simulink model "controladaptable"  (R2023b)
settings: Solver=ode23t  StartTime=0.0  StopTime=25  RelTol=1e-3
values from neighbouring files (symbols this model uses):
  BL = 0.00223579    [ILCadaptable.m]    (also in parametros3.m)
  C1 = [1 0 0 0]    [ILCadaptable.m]    (also in parametros3.m = [1 0 0 0 0 0])
  C2 = [0 1 0 0]    [ILCadaptable.m]    (also in parametros3.m = [0 0 1 0 0 0])
  C3 = [0 0 1 0]    [ILCadaptable.m]    (also in parametros3.m = [0 0 0 0 1 0])
  C4 = [0 0 0 1]    [ILCadaptable.m]
  JL = 0.00040095    [ILCadaptable.m]    (also in parametros3.m)
  KB = 0.23351629    [ILCadaptable.m]    (also in parametros3.m)
  KD = 5    [ILCadaptable.m]
  KM = 0.23351629    [ILCadaptable.m]    (also in parametros3.m)
  LC = 0.0015    [ILCadaptable.m]    (also in parametros3.m)
  RC = 3.4    [ILCadaptable.m]    (also in parametros3.m)
  rt = 10    [ILCadaptable.m]    (also in parametros3.m)
libraries: simulink x2, slpidlib x2
settings Model: Creator=soria  LastModifiedBy=LENOVO
settings SolverCC: AlgebraicLoopSolver=TrustRegion
settings DebuggingCC: UnconnectedInputMsg=warning  UnconnectedOutputMsg=warning  UnconnectedLineMsg=warning
settings ModelReferenceCC: EnableRefExpFcnMdlSchedulingChecks=on

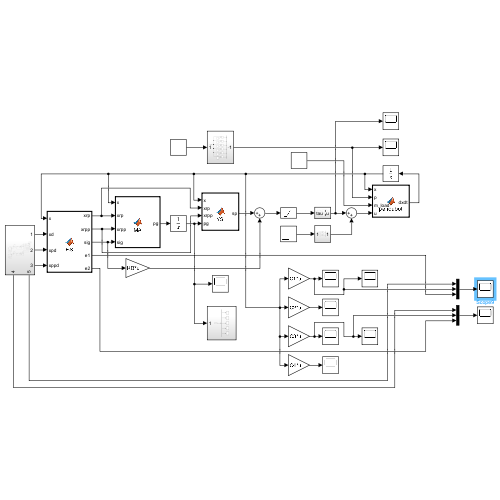
[thumbnail: Simulink's stored preview of the top-level diagram]
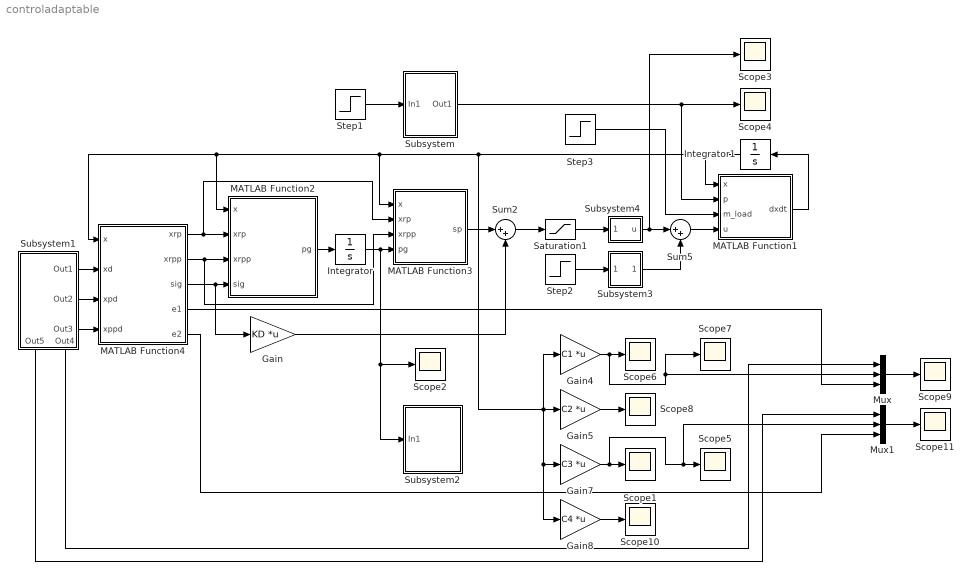
== system controladaptable ==
  Gain : Gain  Gain=KD  Multiplication=Matrix(K*u)
  Gain4 : Gain  Gain=C1  Multiplication=Matrix(K*u)
  Gain5 : Gain  Gain=C2  Multiplication=Matrix(K*u)
  Gain7 : Gain  Gain=C3  Multiplication=Matrix(K*u)
  Gain8 : Gain  Gain=C4  Multiplication=Matrix(K*u)
  Integrator : Integrator  InitialCondition=[0 0 0 0 0]
  Integrator1 : Integrator  InitialCondition=[-pi/2;0;0;0]
  MATLAB Function1 : MATLAB Function  TreatAsAtomicUnit=on
  MATLAB Function2 : MATLAB Function  TreatAsAtomicUnit=on
  MATLAB Function3 : MATLAB Function  TreatAsAtomicUnit=on
  MATLAB Function4 : MATLAB Function  TreatAsAtomicUnit=on
  Mux : Mux  Inputs=3
  Mux1 : Mux  Inputs=3
  Saturation1 : Saturate  UpperLimit=10  LowerLimit=-10
  Scope{1..11} (11 alike) : Scope
  Step1 : Step  Time=0  SampleTime=0
  Step2 : Step  Time=0  After=2  SampleTime=0
  Step3 : Step  Time=10  SampleTime=0
  Subsystem : Subsystem
  Subsystem1 : Subsystem
      settings: PortSchema="{\"entries\":[{\"content\":{\"sides\":[{\"content\":{},\"type\":\"ConnectorPlacement.EquallySpacedRectSide\",\"uuid\":\"9b7d0a68-027c-45ca-820c-f278bc6f32a7\"},{\"content\":{\"connectorIds\":[\"Out1\",\"Out2\",\"Out3\"],\"side\":\"RIGHT\"},\"type\":\"ConnectorPlacement.EquallySpacedRectSide\",\"uuid\":\"fa53ec67-4df6-4868-87ee-3d32a2fc1068\"},{\"content\":{\"side\":\"TOP\"},\"type\":\"ConnectorPlacement.EquallySpacedRectSide\",\"uuid\":\"8fcd41cb-9cc9-4cf7-b08f-50ea27c8effa\"},{\"content\":{\"connectorIds\":[\"Out4\",\"Out5\"],\"side\":\"BOTTOM\"},\"type\":\"ConnectorPlacement.EquallySpacedRectSide\",\"uuid\":\"53ef6b28-bc02-4c26-b41f-4cbf5a6224bd\"}]},\"type\":\"ConnectorPlacement.EquallySpacedConnector\",\"uuid\":\"01489902-74b8-4eba-a27b-b5ca226e6d88\"}],\"packageUris\":[\"http://schema.mathworks.com/mf0/Connector/R2020b\"],\"version\":\"1.0\"}"
  Subsystem2 : Subsystem
  Subsystem3 : Subsystem
  Subsystem4 : Subsystem
  Sum2 : Sum  Inputs=|++
  Sum5 : Sum  Inputs=|++
  wires:
  MATLAB Function2/1(pg) -> Integrator/1
  MATLAB Function4/3(sig) -> Gain/1, MATLAB Function2/4(sig)
  Gain4/1 -> Scope7/1, Mux/2, Scope6/1
  Gain7/1 -> Scope5/1, Mux1/2, Scope1/1
  Gain5/1 -> Scope8/1
  Gain8/1 -> Scope10/1
  MATLAB Function4/2(xrpp) -> MATLAB Function2/3(xrpp), MATLAB Function3/3(xrpp)
  Subsystem1/3(Out3) -> MATLAB Function4/4(xppd)
  Subsystem1/1(Out1) -> MATLAB Function4/2(xd)
  Subsystem1/2(Out2) -> MATLAB Function4/3(xpd)
  Step1/1 -> Subsystem/1(In1)
  Integrator/1 -> Subsystem2/1(In1), Scope2/1, MATLAB Function3/4(pg)
  Integrator1/1 -> MATLAB Function1/1(x), Gain4/1, Gain8/1, Gain7/1, Gain5/1, MATLAB Function2/1(x), MATLAB Function4/1(x), MATLAB Function3/1(x)
  Subsystem/1(Out1) -> Scope4/1, MATLAB Function1/2(p)
  MATLAB Function3/1(sp) -> Sum2/1
  MATLAB Function4/1(xrp) -> MATLAB Function3/2(xrp), MATLAB Function2/2(xrp)
  MATLAB Function1/1(dxdt) -> Integrator1/1
  Mux/1 -> Scope9/1
  Mux1/1 -> Scope11/1
  Subsystem1/5(Out4) -> Mux/1
  Subsystem1/4(Out5) -> Mux1/1
  Subsystem3/1(Out1) -> Sum5/2
  Step2/1 -> Subsystem3/1(In1)
  Gain/1 -> Sum2/2
  Sum5/1 -> MATLAB Function1/4(u)
  Subsystem4/1(u) -> Scope3/1, Sum5/1
  MATLAB Function4/4(e1) -> Mux/3
  MATLAB Function4/5(e2) -> Mux1/3
  Sum2/1 -> Saturation1/1
  Saturation1/1 -> Subsystem4/1(tau)
  Step3/1 -> MATLAB Function1/3(m_load)

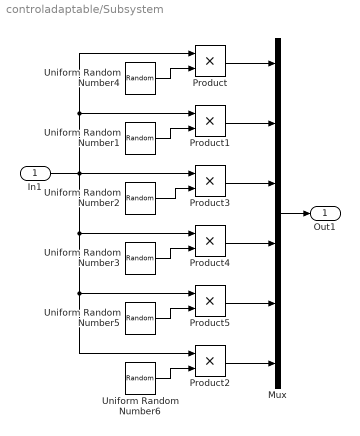
== system controladaptable/Subsystem ==
  In1 : Inport
  Mux : Mux  Inputs=6
  Product{,1..5} (6 alike) : Product
  Uniform Random Number1 : UniformRandomNumber  Minimum=-0.0792  Maximum=0.0792  Seed=2  SampleTime=0.1
  Uniform Random Number2 : UniformRandomNumber  Minimum=-0.025  Maximum=0.025  Seed=1  SampleTime=0.1
  Uniform Random Number3 : UniformRandomNumber  Minimum=-0.03  Maximum=0.03  Seed=3  SampleTime=0.1
  Uniform Random Number4 : UniformRandomNumber  Minimum=-0.066  Maximum=0.066  SampleTime=0.1
  Uniform Random Number5 : UniformRandomNumber  Minimum=-0.00138  Maximum=0.00138  Seed=1.5  SampleTime=0.1
  Uniform Random Number6 : UniformRandomNumber  Minimum=-0.00238  Maximum=0.00238  Seed=1.5  SampleTime=0.1
  Out1 : Outport
  wires:
  Product/1 -> Mux/1
  Uniform Random Number5/1 -> Product5/2
  Uniform Random Number1/1 -> Product1/2
  In1/1 -> Product2/1, Product5/1, Product4/1, Product3/1, Product/1, Product1/1
  Uniform Random Number2/1 -> Product3/2
  Product4/1 -> Mux/4
  Product1/1 -> Mux/2
  Uniform Random Number3/1 -> Product4/2
  Uniform Random Number4/1 -> Product/2
  Product3/1 -> Mux/3
  Product5/1 -> Mux/5
  Mux/1 -> Out1/1
  Product2/1 -> Mux/6
  Uniform Random Number6/1 -> Product2/2

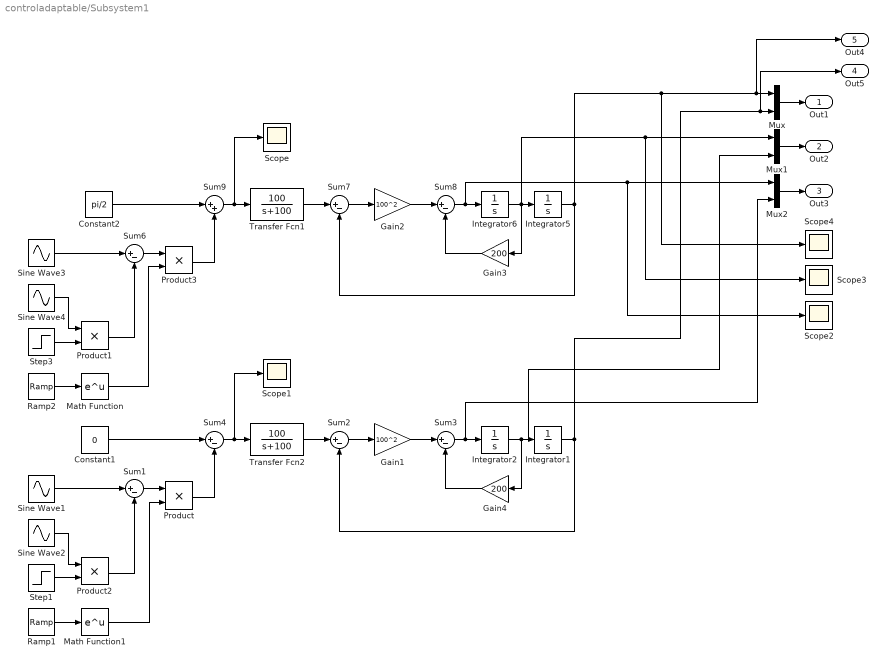
== system controladaptable/Subsystem1 ==
  Constant1 : Constant  Value=0
  Constant2 : Constant  Value=pi/2
  Gain1 : Gain  Gain=100^2
  Gain2 : Gain  Gain=100^2
  Gain3 : Gain  Gain=200
  Gain4 : Gain  Gain=200
  Integrator{1..2,5..6} (4 alike) : Integrator
  Math Function : Math
  Math Function1 : Math
  Mux : Mux  Inputs=2
  Mux1 : Mux  Inputs=2
  Mux2 : Mux  Inputs=2
  Product{,1..3} (4 alike) : Product
  Ramp1 : simulink/Sources/Ramp  slope=0  start=10  InitialOutput=0
  Ramp2 : simulink/Sources/Ramp  slope=0  start=10  InitialOutput=0
  Scope{,1..4} (5 alike) : Scope
  Sine Wave1 : Sin  Amplitude=1.4  Frequency=2  SampleTime=0
  Sine Wave2 : Sin  Amplitude=1.4  Frequency=5  SampleTime=0
  Sine Wave3 : Sin  Amplitude=1.4  Frequency=2  SampleTime=0
  Sine Wave4 : Sin  Amplitude=1.4  Frequency=5  SampleTime=0
  Step1 : Step  Time=0  After=0  SampleTime=0
  Step3 : Step  Time=0  After=0  SampleTime=0
  Sum{1..4,6..8} (7 alike) : Sum  Inputs=|+-
  Sum9 : Sum  Inputs=|++
  Transfer Fcn1 : TransferFcn  Numerator=[100]  Denominator=[1 100]
  Transfer Fcn2 : TransferFcn  Numerator=[100]  Denominator=[1 100]
  Out1 : Outport
  Out2 : Outport  Port=2
  Out3 : Outport  Port=3
  Out5 : Outport  Port=4
  Out4 : Outport  Port=5
  wires:
  Mux/1 -> Out1/1
  Mux1/1 -> Out2/1
  Mux2/1 -> Out3/1
  Integrator5/1 -> Scope4/1, Out4/1, Mux/1, Sum7/2
  Sine Wave3/1 -> Sum6/1
  Sum7/1 -> Gain2/1
  Sum8/1 -> Scope2/1, Mux2/1, Integrator6/1
  Sine Wave4/1 -> Product1/1
  Gain2/1 -> Sum8/1
  Transfer Fcn1/1 -> Sum7/1
  Gain3/1 -> Sum8/2
  Product1/1 -> Sum6/2
  Step3/1 -> Product1/2
  Constant2/1 -> Sum9/1
  Integrator6/1 -> Scope3/1, Mux1/1, Gain3/1, Integrator5/1
  Sum9/1 -> Scope/1, Transfer Fcn1/1
  Sum4/1 -> Scope1/1, Transfer Fcn2/1
  Sum3/1 -> Mux2/2, Integrator2/1
  Gain1/1 -> Sum3/1
  Transfer Fcn2/1 -> Sum2/1
  Sum2/1 -> Gain1/1
  Step1/1 -> Product2/2
  Constant1/1 -> Sum4/1
  Integrator1/1 -> Out5/1, Mux/2, Sum2/2
  Sine Wave1/1 -> Sum1/1
  Gain4/1 -> Sum3/2
  Integrator2/1 -> Mux1/2, Gain4/1, Integrator1/1
  Product2/1 -> Sum1/2
  Sine Wave2/1 -> Product2/1
  Math Function/1 -> Product3/2
  Math Function1/1 -> Product/2
  Ramp2/1 -> Math Function/1
  Ramp1/1 -> Math Function1/1
  Sum6/1 -> Product3/1
  Product3/1 -> Sum9/2
  Sum1/1 -> Product/1
  Product/1 -> Sum4/2

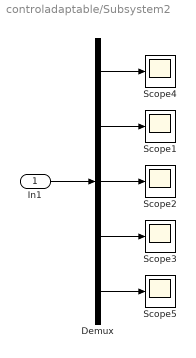
== system controladaptable/Subsystem2 ==
  In1 : Inport
  Demux : Demux  Outputs=5
  Scope{1..5} (5 alike) : Scope
  wires:
  In1/1 -> Demux/1
  Demux/3 -> Scope2/1
  Demux/2 -> Scope1/1
  Demux/1 -> Scope4/1
  Demux/4 -> Scope3/1
  Demux/5 -> Scope5/1

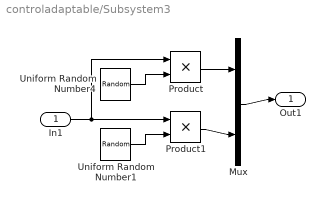
== system controladaptable/Subsystem3 ==
  In1 : Inport
  Mux : Mux  Inputs=2
  Product : Product
  Product1 : Product
  Uniform Random Number1 : UniformRandomNumber  Seed=2  SampleTime=0.1
  Uniform Random Number4 : UniformRandomNumber  SampleTime=0.1
  Out1 : Outport
  wires:
  Product/1 -> Mux/1
  Uniform Random Number1/1 -> Product1/2
  In1/1 -> Product/1, Product1/1
  Product1/1 -> Mux/2
  Uniform Random Number4/1 -> Product/2
  Mux/1 -> Out1/1

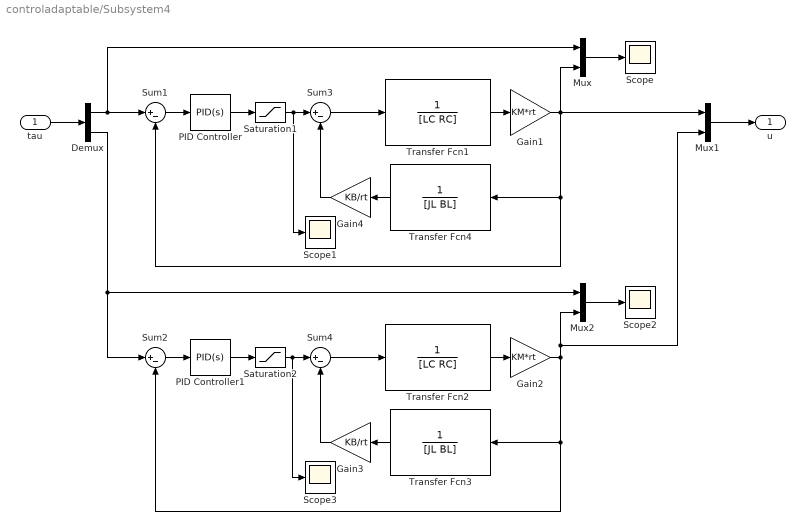
== system controladaptable/Subsystem4 ==
  tau : Inport
  Demux : Demux  Outputs=2
  Gain1 : Gain  Gain=KM*rt
  Gain2 : Gain  Gain=KM*rt
  Gain3 : Gain  Gain=KB/rt
  Gain4 : Gain  Gain=KB/rt
  Mux : Mux  Inputs=2
  Mux1 : Mux  Inputs=2
  Mux2 : Mux  Inputs=2
  PID Controller : slpidlib/PID Controller  Controller=PID  Form=Parallel  TimeDomain=Continuous-time  UseExternalTs=off  SampleTime=-1  IntegratorMethod=Forward Euler  FilterMethod=Forward Euler  ControllerParametersSource=internal  P=100  I=50  UseKiTs=off  D=20  N=100  UseFilter=on  TunerSelectOption=Transfer Function Based (PID Tuner App)  InitialConditionSource=internal  InitialConditionForIntegrator=0  InitialConditionForFilter=0  DifferentiatorICPrevScaledInput=0  ExternalReset=none  TrackingMode=off  Kt=1  LimitOutput=off  SatLimitsSource=internal  UpperSaturationLimit=inf  LowerSaturationLimit=-inf  LinearizeAsGain=on  AntiWindupMode=none  Kb=1  LimitIntegrator=off  UpperIntegratorSaturationLimit=inf  LowerIntegratorSaturationLimit=-inf  POutMin=[]  POutMax=[]  IOutMin=[]  IOutMax=[]  DOutMin=[]  DOutMax=[]  NOutMin=[]  NOutMax=[]  SumOutMin=[]  SumOutMax=[]  SaturationOutMin=[]  SaturationOutMax=[]  PParamMin=[]  PParamMax=[]  IParamMin=[]  IParamMax=[]  DParamMin=[]  DParamMax=[]  NParamMin=[]  NParamMax=[]  KbParamMin=[]  KbParamMax=[]  KtParamMin=[]  KtParamMax=[]  KbOutMin=[]  KbOutMax=[]  KtOutMin=[]  KtOutMax=[]  IntegratorOutMin=[]  IntegratorOutMax=[]  FilterOutMin=[]  FilterOutMax=[]  SumI1OutMin=[]  SumI1OutMax=[]  SumI2OutMin=[]  SumI2OutMax=[]  SumI3OutMin=[]  SumI3OutMax=[]  SumI4OutMin=[]  SumI4OutMax=[]  SumDOutMin=[]  SumDOutMax=[]  DifferentiatorOutMin=[]  DifferentiatorOutMax=[]  FilterDiffOutCoefMin=[]  FilterDiffOutCoefMax=[]  ReciprocalOutMin=[]  ReciprocalOutMax=[]  SumDenOutMin=[]  SumDenOutMax=[]  SumNumOutMin=[]  SumNumOutMax=[]  DivideOutMin=[]  DivideOutMax=[]  UdiffTsProdOutMin=[]  UdiffTsProdOutMax=[]  NTsProdOutMin=[]  NTsProdOutMax=[]  UintegralTsProdOutMin=[]  UintegralTsProdOutMax=[]  UngainTsProdOutMin=[]  UngainTsProdOutMax=[]  ClampingZeroOutDataTypeStr=Inherit: Inherit via back propagation  ClampingZeroOutMin=[]  ClampingZeroOutMax=[]  FilterDenConstantOutDataTypeStr=Inherit: Inherit via back propagation  FilterDenConstantOutMin=[]  FilterDenConstantOutMax=[]  PCopyOutDataTypeStr=Inherit: Inherit via back propagation  PCopyOutMin=[]  PCopyOutMax=[]  NCopyOutDataTypeStr=Inherit: Inherit via back propagation  NCopyOutMin=[]  NCopyOutMax=[]  IntegratorContinuousStateAttributes=''  IntegratorStateMustResolveToSignalObject=off  IntegratorRTWStateStorageClass=Auto  FilterContinuousStateAttributes=''  FilterStateMustResolveToSignalObject=off  FilterRTWStateStorageClass=Auto  ParallelPVariant=InternalParameters  IdealPVariant=Disabled  IVariant=InternalParameters  DVariant=InternalParameters  IntegratorVariant=Continuous  SatVariant=Disabled  AWVariant=Passthrough  PCopyVariant=Disabled  TRVariant=Disabled  FdbkBlocksVariant=Forward  IdealPFdbkVariant=Disabled  SatFdbkVariant=Disabled  DerivativeFilterVariant=ContFilter  NVariant=InternalParameters  NCopyVariant=Disabled  FilterICVariant=InternalICsFilter  IntegratorICVariant=InternalICs  ExternalResetVariant=Disabled  TRSumVariant=Passthrough  SumFdbkVariant=Disabled  SumVariant=Sum_PID  TsampFilterVariant=InternalTs  TsampNgainVariant=Passthrough  TsampIntegralVariant=Disabled_SignalSpec  ExternalSaturationOutDataTypeStr=Inherit: Same as second input
  PID Controller1 : slpidlib/PID Controller  Controller=PID  Form=Parallel  TimeDomain=Continuous-time  UseExternalTs=off  SampleTime=-1  IntegratorMethod=Forward Euler  FilterMethod=Forward Euler  ControllerParametersSource=internal  P=100  I=50  UseKiTs=off  D=20  N=100  UseFilter=on  TunerSelectOption=Transfer Function Based (PID Tuner App)  InitialConditionSource=internal  InitialConditionForIntegrator=0  InitialConditionForFilter=0  DifferentiatorICPrevScaledInput=0  ExternalReset=none  TrackingMode=off  Kt=1  LimitOutput=off  SatLimitsSource=internal  UpperSaturationLimit=inf  LowerSaturationLimit=-inf  LinearizeAsGain=on  AntiWindupMode=none  Kb=1  LimitIntegrator=off  UpperIntegratorSaturationLimit=inf  LowerIntegratorSaturationLimit=-inf  POutMin=[]  POutMax=[]  IOutMin=[]  IOutMax=[]  DOutMin=[]  DOutMax=[]  NOutMin=[]  NOutMax=[]  SumOutMin=[]  SumOutMax=[]  SaturationOutMin=[]  SaturationOutMax=[]  PParamMin=[]  PParamMax=[]  IParamMin=[]  IParamMax=[]  DParamMin=[]  DParamMax=[]  NParamMin=[]  NParamMax=[]  KbParamMin=[]  KbParamMax=[]  KtParamMin=[]  KtParamMax=[]  KbOutMin=[]  KbOutMax=[]  KtOutMin=[]  KtOutMax=[]  IntegratorOutMin=[]  IntegratorOutMax=[]  FilterOutMin=[]  FilterOutMax=[]  SumI1OutMin=[]  SumI1OutMax=[]  SumI2OutMin=[]  SumI2OutMax=[]  SumI3OutMin=[]  SumI3OutMax=[]  SumI4OutMin=[]  SumI4OutMax=[]  SumDOutMin=[]  SumDOutMax=[]  DifferentiatorOutMin=[]  DifferentiatorOutMax=[]  FilterDiffOutCoefMin=[]  FilterDiffOutCoefMax=[]  ReciprocalOutMin=[]  ReciprocalOutMax=[]  SumDenOutMin=[]  SumDenOutMax=[]  SumNumOutMin=[]  SumNumOutMax=[]  DivideOutMin=[]  DivideOutMax=[]  UdiffTsProdOutMin=[]  UdiffTsProdOutMax=[]  NTsProdOutMin=[]  NTsProdOutMax=[]  UintegralTsProdOutMin=[]  UintegralTsProdOutMax=[]  UngainTsProdOutMin=[]  UngainTsProdOutMax=[]  ClampingZeroOutDataTypeStr=Inherit: Inherit via back propagation  ClampingZeroOutMin=[]  ClampingZeroOutMax=[]  FilterDenConstantOutDataTypeStr=Inherit: Inherit via back propagation  FilterDenConstantOutMin=[]  FilterDenConstantOutMax=[]  PCopyOutDataTypeStr=Inherit: Inherit via back propagation  PCopyOutMin=[]  PCopyOutMax=[]  NCopyOutDataTypeStr=Inherit: Inherit via back propagation  NCopyOutMin=[]  NCopyOutMax=[]  IntegratorContinuousStateAttributes=''  IntegratorStateMustResolveToSignalObject=off  IntegratorRTWStateStorageClass=Auto  FilterContinuousStateAttributes=''  FilterStateMustResolveToSignalObject=off  FilterRTWStateStorageClass=Auto  ParallelPVariant=InternalParameters  IdealPVariant=Disabled  IVariant=InternalParameters  DVariant=InternalParameters  IntegratorVariant=Continuous  SatVariant=Disabled  AWVariant=Passthrough  PCopyVariant=Disabled  TRVariant=Disabled  FdbkBlocksVariant=Forward  IdealPFdbkVariant=Disabled  SatFdbkVariant=Disabled  DerivativeFilterVariant=ContFilter  NVariant=InternalParameters  NCopyVariant=Disabled  FilterICVariant=InternalICsFilter  IntegratorICVariant=InternalICs  ExternalResetVariant=Disabled  TRSumVariant=Passthrough  SumFdbkVariant=Disabled  SumVariant=Sum_PID  TsampFilterVariant=InternalTs  TsampNgainVariant=Passthrough  TsampIntegralVariant=Disabled_SignalSpec  ExternalSaturationOutDataTypeStr=Inherit: Same as second input
  Saturation1 : Saturate  UpperLimit=250  LowerLimit=-250
  Saturation2 : Saturate  UpperLimit=250  LowerLimit=-250
  Scope{,1..3} (4 alike) : Scope
  Sum{1..4} (4 alike) : Sum  Inputs=|+-
  Transfer Fcn1 : TransferFcn  Denominator=[LC RC]
  Transfer Fcn2 : TransferFcn  Denominator=[LC RC]
  Transfer Fcn3 : TransferFcn  Denominator=[JL BL]
  Transfer Fcn4 : TransferFcn  Denominator=[JL BL]
  u : Outport
  wires:
  tau/1 -> Demux/1
  Demux/1 -> Sum1/1, Mux/1
  Mux/1 -> Scope/1
  Sum1/1 -> PID Controller/1
  Transfer Fcn1/1 -> Gain1/1
  Gain1/1 -> Sum1/2, Transfer Fcn4/1, Mux1/1, Mux/2
  Gain4/1 -> Sum3/2
  Sum3/1 -> Transfer Fcn1/1
  Transfer Fcn4/1 -> Gain4/1
  Mux1/1 -> u/1
  PID Controller/1 -> Saturation1/1
  PID Controller1/1 -> Saturation2/1
  Sum2/1 -> PID Controller1/1
  Demux/2 -> Sum2/1, Mux2/1
  Transfer Fcn2/1 -> Gain2/1
  Transfer Fcn3/1 -> Gain3/1
  Gain3/1 -> Sum4/2
  Gain2/1 -> Mux2/2, Mux1/2, Sum2/2, Transfer Fcn3/1
  Mux2/1 -> Scope2/1
  Sum4/1 -> Transfer Fcn2/1
  Saturation1/1 -> Scope1/1, Sum3/1
  Saturation2/1 -> Scope3/1, Sum4/1

== matlab function controladaptable/MATLAB Function1 ==
  data: x input; p input; m_load input; u input; dxdt output
function dxdt = pendubot(x,p,m_load,u)

%definición de parametros
m1 = 0.066+p(1)+m_load;
m2 = 0.0792+p(2);
l1 = 0.25+p(3);
l2 = 0.3+p(4);
lc1 = l1/2;
lc2 = l2/2;
I1 = 0.00138+p(5);
I2 = 0.00238+p(6);
g = 9.81;

%calculo de las constantes del sistema
a1 = m1*lc1^2+m2*l1^2+I1;
a2 = m2*lc2^2+I2;
a3 = m2*l1*lc2;
a4 = m1*lc1+m2*l1;
a5 = m2*lc2;

%variables de estado
x1 = x(1);
x2 = x(2);
x3 = x(3);
x4 = x(4);

%Matrices del sistema
G = [a4*g*cos(x1)+a5*g*cos(x1+x3);a5*g*cos(x1+x3)];%matriz de gravedad 
C = [-2*a3*sin(x3)*x4 -a3*sin(x3)*x4;
     a3*sin(x3)*x2 0];%matriz de velocidad o coriolis
M = [a1+a2+2*a3*cos(x3) a2+a3*cos(x3);
     a2+a3*cos(x3) a2];%matriz de aceleración

%d/dt[x1;x2;x3;x4]=[f1;f2;f3;f4]
%calculo de f2 y f4 
xb = M^(-1)*u-M^(-1)*C*[x2;x4]-M^(-1)*G;

%sistema en la forma d/dt[x1;x2;x3;x4]=[f1;f2;f3;f4] 
dxdt = [x2; 
        xb(1);
        x4;
        xb(2)];

== matlab function controladaptable/MATLAB Function3 ==
  data: x input; xrp input; xrpp input; pg input; sp output
function sp = YS(x,xrp,xrpp,pg)

%variables de estado
x1 = x(1);
x2 = x(2);
x3 = x(3);
x4 = x(4);

%Matriz Y(x,xr) equivalente
Y = [xrpp(1),xrpp(1)+xrpp(2),cos(x3)*xrpp(1)+cos(x3)*xrpp(2)-2*sin(x3)*x4*xrp(1)-sin(x3)*x4*xrp(2),cos(x3),cos(x1+x3);0,xrpp(1)+xrpp(2),cos(x3)*xrpp(1)+sin(x3)*x2*xrp(1),0,cos(x1+x3)];

%acción de control final
sp = Y*pg

== matlab function controladaptable/MATLAB Function2 ==
  data: x input; xrp input; xrpp input; sig input; pg output
function pg = MA(x,xrp,xrpp,sig)

%variables de estado
x1 = x(1);
x2 = x(2);
x3 = x(3);
x4 = x(4);

%Matriz Y(x,xr) equivalente
Y = [xrpp(1),xrpp(1)+xrpp(2),cos(x3)*xrpp(1)+cos(x3)*xrpp(2)-2*sin(x3)*x4*xrp(1)-sin(x3)*x4*xrp(2),cos(x3),cos(x1+x3);0,xrpp(1)+xrpp(2),cos(x3)*xrpp(1)+sin(x3)*x2*xrp(1),0,cos(x1+x3)];

%Ganancia Kpi de parametros
Kpi = 10000*[1 0 0 0 0;0 1 0 0 0;0 0 1 0 0;0 0 0 1 0;0 0 0 0 1]

%acción de control
pg = Kpi^(-1)*Y'*sig

== matlab function controladaptable/MATLAB Function4 ==
  data: x input; xd input; xpd input; xppd input; xrp output; xrpp output; sig output; e1 output; e2 output
function [xrp,xrpp,sig,e1,e2] = ES(x,xd,xpd,xppd)

%variables de estado
xp = [x(1);x(3)];
xv = [x(2);x(4)];

%Ganancia del error de segumiento
A = 2*[1 0;0 1];

%Calculo de velocidad y aceleración de referencia
xg = xd-xp;
xgp = xpd-xv;
e1 = xg(1);
e2 = xg(2);

xrp = xpd+A*xg;
xrpp = xppd+A*xgp;

%error de seguimiento
sig = xrp-xv
